simulink model "regler"  (Simulink 7.9)
settings: Solver=ode3  StartTime=0.0  StopTime=10  FixedStep=0.01  MaxStep=1e-3  RelTol=1e-3
PreLoadFcn:
  | l=0.23 %Achsenlänge in m
  | mc=0.5 %Masse Chassis in kg
  | mm=0.02 %Masse einzelner Motor in Kg
  | J=(l^2)*0.5*((1/12)*mc+mm)%Trägheitmoment rollen+nicken
  | Jg=(1/12)*mc*(l^2)+mm*4*(l/2)^2%trägheitsmoment gieren
  | tau=1/16.28; %zeitkonstante pt1-glied
  | k=2.064e+04; %proportionalitätsfaktor pt1glied
  | mi_wurz=-(sqrt(2)/2)*l/2; %initwerte
  | plu_wurz=(sqrt(2)/2)*l/2; %initwerte
  | mges=0.5 %Gesamtmasse in kg
  | %Drehmomentfunktion
  | %Funktion M(n) AUfstellen
  | kt=0.415*1e-2; %Nm/A
  | p1=[1.4 , 25000];
  | p2=[15.5 , 15000];
  | m=(p2(2)-p1(2))/(p2(1)-p1(1));
  | c=p1(2)-m*p1(1);
  | mm=kt/m;
  | cm=(-1)*c*mm;
  | %Propeller Funktion
  | faktor = 0.8895305;
  | exponent = 2.015137;
  | 
  | %regelparameter
  | kp_roll=0.75
  | tn_roll=1000
  | tv_roll=1.5
  | tp_roll=0.04
  | kp_v_roll=5.8571
  | kp_a_roll=0.0070
  | 
  | kp_nick=0.75
  | tn_nick=1000
  | tv_nick=1.5
  | tp_nick=0.04
  | kp_v_nick=5.8571
  | kp_a_nick=0.0070
  | 
  | kp_gier=0.75
  | tn_gier=1000
  | tv_gier=1.5
  | tp_gier=0.04
  | kp_v_gier=5.8571
  | kp_a_gier=0.0070
  | 
  | %Motor skalierungsfaktor
  | k_motor_out=1;
  | %maximaldrehzahl Motor
  | n_max=20000;
libraries: simulink x4, aerolibutil x4
settings Model: Creator=Flo  LastModifiedBy=Flo  TunableVars=exponent,faktor,k_motor_out,kp_a_gier,kp_a_nick,kp_a_roll,kp_gier,kp_nick,kp_roll,kp_v_gier,kp_v_nick,kp_v_roll,n_max,tn_gier,tn_nick,tn_roll,tp_gier,tp_nick,tp_roll,tv_gier,tv_nick,tv_roll  TunableVarsStorageClass=ExportedGlobal,ExportedGlobal,ExportedGlobal,ExportedGlobal,ExportedGlobal,ExportedGlobal,ExportedGlobal,ExportedGlobal,ExportedGlobal,ExportedGlobal,ExportedGlobal,ExportedGlobal,ExportedGlobal,ExportedGlobal,ExportedGlobal,ExportedGlobal,ExportedGlobal,ExportedGlobal,ExportedGlobal,ExportedGlobal,ExportedGlobal,ExportedGlobal  TunableVarsTypeQualifier=,,,,,,,,,,,,,,,,,,,,,
settings OptimizationCC: InlineParams=on  UseSpecifiedMinMax=on  EnableMemcpy=off  PassReuseOutputArgsAs=Individual arguments  OptimizeModelRefInitCode=on  LifeSpan=1
settings RTWCC: SystemTargetFile=ert.tlc  TemplateMakefile=ert_default_tmf  Description=Embedded Coder  ProcessScript=ert_make_rtw_hook  TargetLang=C++  RTWCompilerOptimization=On  CheckMdlBeforeBuild=Warning
settings CodeAppCC: IgnoreCustomStorageClasses=off
settings ERTTargetCC: CodeReplacementLibrary=C89/C90 (ANSI)  ERTMultiwordTypeDef=User defined  MultiwordLength=2048  GenerateSampleERTMain=on  SupportComplex=off  SupportContinuousTime=on  ERTCustomFileTemplate=example_file_process.tlc  GlobalDataDefinition=InSourceFile  DataDefinitionFile=.c  GlobalDataReference=InSourceFile  ConvertIfToSwitch=off  SuppressUnreachableDefaultCases=off  EnableUserReplacementTypes=on

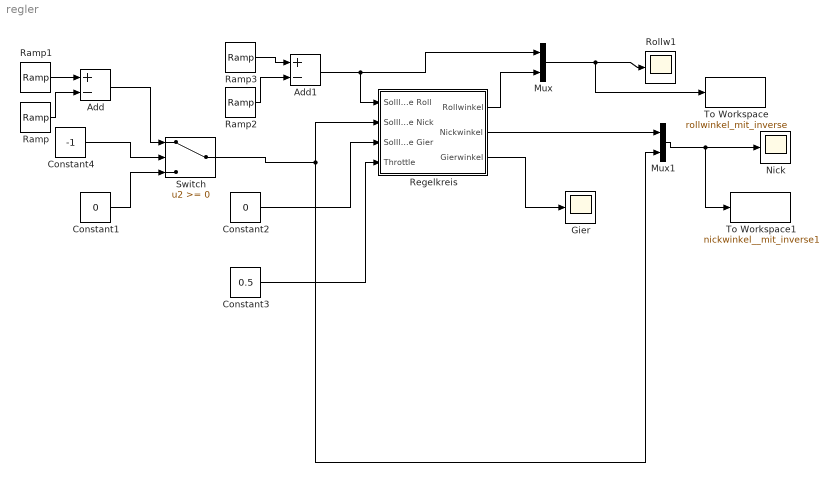
== system regler ==
  Add : Sum  Inputs=+-
  Add1 : Sum  Inputs=+-
  Constant1 : Constant  Value=0
  Constant2 : Constant  Value=0
  Constant3 : Constant  Value=0.5
  Constant4 : Constant  Value=-1
  Gier : Scope
      settings: YMin=0.05  YMax=0.275  SaveName=ScopeData25
  Mux : Mux  Inputs=2
  Mux1 : Mux  Inputs=2
  Nick : Scope
      settings: YMin=0.8  YMax=0.94  SaveName=ScopeData26
  Ramp : simulink/Sources/Ramp  slope=4  start=1.05  X0=0
  Ramp1 : simulink/Sources/Ramp  slope=4  start=1  X0=0
  Ramp2 : simulink/Sources/Ramp  slope=4  start=1.6  X0=0
  Ramp3 : simulink/Sources/Ramp  slope=4  start=1.5  X0=0
  Regelkreis : Subsystem
  Rollw1 : Scope
      settings: TimeRange=0.03425507699014805  YMin=0.5004659956947598  YMax=0.5014065398919517  SaveName=ScopeData2
  Switch : Switch
  To Workspace : ToWorkspace  VariableName=rollwinkel_mit_inverse  SampleTime=-1  SaveFormat=Timeseries
  To Workspace1 : ToWorkspace  VariableName=nickwinkel__mit_inverse1  SampleTime=-1  SaveFormat=Timeseries
  wires:
  Constant2/1 -> Regelkreis/3(Solllage Gier)
  Constant3/1 -> Regelkreis/4(Throttle)
  Regelkreis/1(Rollwinkel) -> Mux/2
  Regelkreis/3(Gierwinkel) -> Gier/1
  Ramp1/1 -> Add/1
  Ramp/1 -> Add/2
  Mux/1 -> Rollw1/1, To Workspace/1
  Add/1 -> Switch/1
  Constant4/1 -> Switch/2
  Ramp3/1 -> Add1/1
  Ramp2/1 -> Add1/2
  Switch/1 -> Regelkreis/2(Solllage Nick), Mux1/2
  Mux1/1 -> Nick/1, To Workspace1/1
  Regelkreis/2(Nickwinkel) -> Mux1/1
  Constant1/1 -> Switch/3
  Add1/1 -> Mux/1, Regelkreis/1(Solllage Roll)

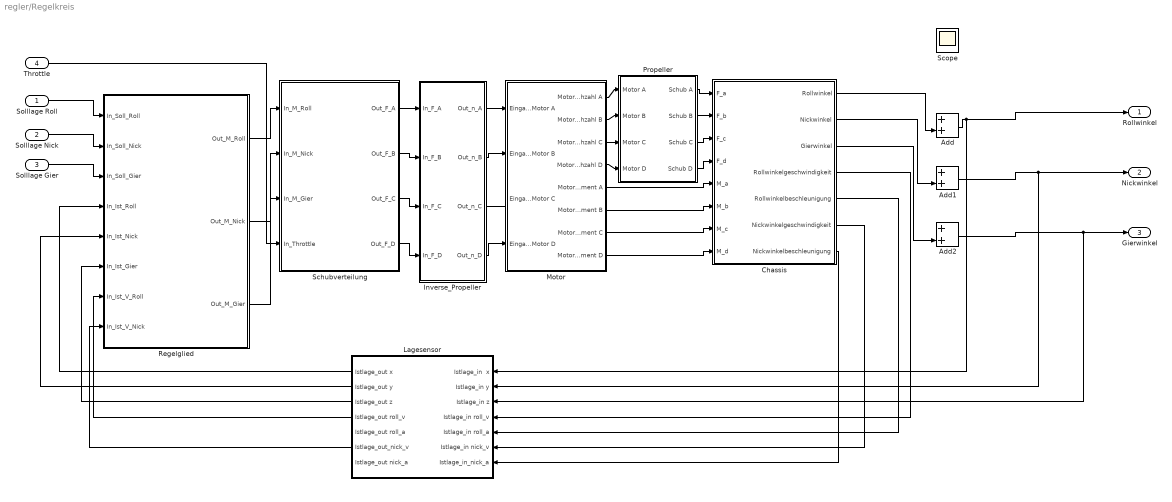
== system regler/Regelkreis ==
  Solllage Roll : Inport
  Solllage Nick : Inport  Port=2
  Solllage Gier : Inport  Port=3
  Throttle : Inport  Port=4
  Add : Sum
  Add1 : Sum
  Add2 : Sum
  Chassis : Subsystem
  Inverse_Propeller : Subsystem
  Lagesensor : Subsystem
  Motor : Subsystem
  Propeller : Subsystem
  Regelglied : Subsystem
  Schubverteilung : Subsystem
  Scope : Scope
      settings: SaveName=ScopeData5
  Rollwinkel : Outport
  Nickwinkel : Outport  Port=2
  Gierwinkel : Outport  Port=3
  wires:
  Motor/1(Motordrehzahl A) -> Propeller/1(Motor A)
  Motor/2(" Motordrehzahl B") -> Propeller/2(Motor B)
  Motor/3(Motordrehzahl C) -> Propeller/3(Motor C)
  Motor/4(Motordrehzahl D) -> Propeller/4(Motor D)
  Propeller/1(Schub A) -> Chassis/1(F_a)
  Propeller/2(Schub B) -> Chassis/2(F_b)
  Propeller/3(Schub C) -> Chassis/3(F_c)
  Propeller/4(Schub D) -> Chassis/4(F_d)
  Motor/5(Motormoment A) -> Chassis/5(M_a)
  Motor/6(" Motormoment B") -> Chassis/6(M_b)
  Motor/7(Motormoment C) -> Chassis/7(M_c)
  Motor/8(Motormoment D) -> Chassis/8(M_d)
  Solllage Roll/1 -> Regelglied/1(In_Soll_Roll)
  Solllage Nick/1 -> Regelglied/2(In_Soll_Nick)
  Solllage Gier/1 -> Regelglied/3(In_Soll_Gier)
  Lagesensor/1(Istlage_out x) -> Regelglied/4(In_Ist_Roll)
  Lagesensor/2(Istlage_out y) -> Regelglied/5(In_Ist_Nick)
  Lagesensor/3(Istlage_out z) -> Regelglied/6(In_Ist_Gier)
  Chassis/2(Nickwinkel) -> Add1/2
  Chassis/1(Rollwinkel) -> Add/2
  Chassis/3(Gierwinkel) -> Add2/2
  Add/1 -> Rollwinkel/1, Lagesensor/1(Istlage_in  x)
  Add1/1 -> Nickwinkel/1, Lagesensor/2(Istlage_in y)
  Add2/1 -> Gierwinkel/1, Lagesensor/3(Istlage_in z)
  ? -> Add1/1, Add2/1, Add/1, Scope/1
  Regelglied/1(Out_M_Roll) -> Schubverteilung/1(In_M_Roll)
  Regelglied/2(Out_M_Nick) -> Schubverteilung/2(In_M_Nick)
  Regelglied/3(Out_M_Gier) -> Schubverteilung/3(In_M_Gier)
  Chassis/4(Rollwinkelgeschwindigkeit) -> Lagesensor/4(Istlage_in roll_v)
  Lagesensor/4(Istlage_out roll_v) -> Regelglied/7(In_Ist_V_Roll)
  Chassis/5(Rollwinkelbeschleunigung) -> Lagesensor/5(Istlage_in roll_a)
  Chassis/6(Nickwinkelgeschwindigkeit) -> Lagesensor/6(Istlage_in nick_v)
  Chassis/7(Nickwinkelbeschleunigung) -> Lagesensor/7(Istlage_in_nick_a)
  Lagesensor/6(Istlage_out_nick_v) -> Regelglied/8(In_Ist_V_Nick)
  Schubverteilung/1(Out_F_A) -> Inverse_Propeller/1(In_F_A)
  Schubverteilung/2(Out_F_B) -> Inverse_Propeller/2(In_F_B)
  Schubverteilung/3(Out_F_C) -> Inverse_Propeller/3(In_F_C)
  Schubverteilung/4(Out_F_D) -> Inverse_Propeller/4(In_F_D)
  Inverse_Propeller/1(Out_n_A) -> Motor/1(Eingang Motor A)
  Inverse_Propeller/2(Out_n_B) -> Motor/2(Eingang Motor B)
  Inverse_Propeller/3(Out_n_C) -> Motor/3(Eingang Motor C)
  Inverse_Propeller/4(Out_n_D) -> Motor/4(Eingang Motor D)
  Throttle/1 -> Schubverteilung/4(In_Throttle)

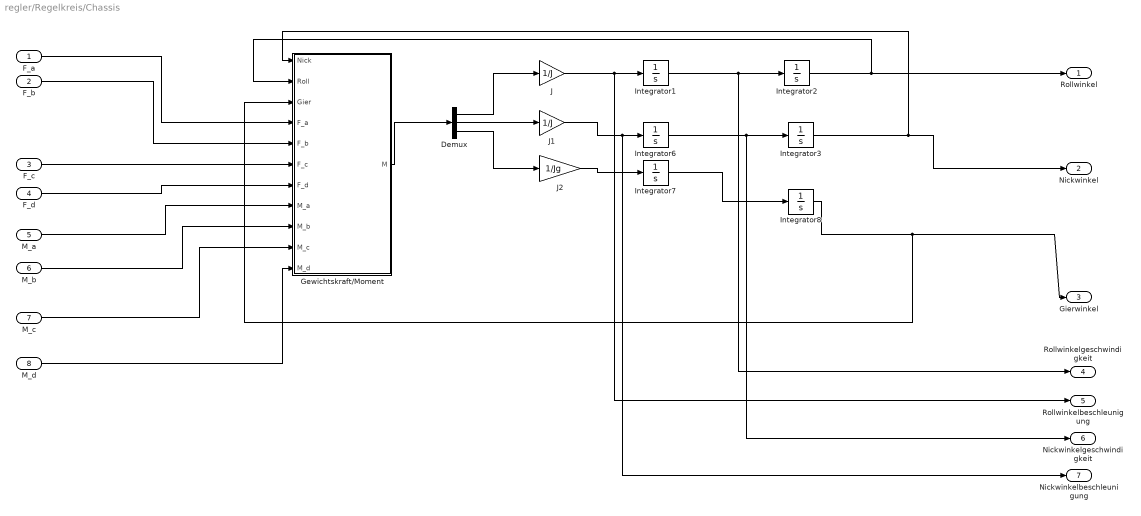
== system regler/Regelkreis/Chassis ==
  F_a : Inport
  F_b : Inport  Port=2
  F_c : Inport  Port=3
  F_d : Inport  Port=4
  M_a : Inport  Port=5
  M_b : Inport  Port=6
  M_c : Inport  Port=7
  M_d : Inport  Port=8
  Demux : Demux  Outputs=3
  Gewichtskraft/Moment : Subsystem
  Integrator{1..3,6..8} (6 alike) : Integrator
  J : Gain  Gain=1/J
  J1 : Gain  Gain=1/J
  J2 : Gain  Gain=1/Jg
  Rollwinkel : Outport
  Nickwinkel : Outport  Port=2
  Gierwinkel : Outport  Port=3
  Rollwinkelgeschwindigkeit : Outport  Port=4
  Rollwinkelbeschleunigung : Outport  Port=5
  Nickwinkelgeschwindigkeit : Outport  Port=6
  Nickwinkelbeschleunigung : Outport  Port=7
  wires:
  F_a/1 -> Gewichtskraft/Moment/4(F_a)
  F_b/1 -> Gewichtskraft/Moment/5(F_b)
  F_c/1 -> Gewichtskraft/Moment/6(F_c)
  F_d/1 -> Gewichtskraft/Moment/7(F_d)
  Gewichtskraft/Moment/1(M) -> Demux/1
  Demux/1 -> J/1
  Demux/2 -> J1/1
  Demux/3 -> J2/1
  J/1 -> Integrator1/1, Rollwinkelbeschleunigung/1
  Integrator1/1 -> Integrator2/1, Rollwinkelgeschwindigkeit/1
  Integrator2/1 -> Rollwinkel/1, Gewichtskraft/Moment/2(Roll)
  J1/1 -> Integrator6/1, Nickwinkelbeschleunigung/1
  Integrator6/1 -> Integrator3/1, Nickwinkelgeschwindigkeit/1
  Integrator3/1 -> Nickwinkel/1, Gewichtskraft/Moment/1(Nick)
  J2/1 -> Integrator7/1
  Integrator7/1 -> Integrator8/1
  Integrator8/1 -> Gierwinkel/1, Gewichtskraft/Moment/3(Gier)
  M_a/1 -> Gewichtskraft/Moment/8(M_a)
  M_b/1 -> Gewichtskraft/Moment/9(M_b)
  M_c/1 -> Gewichtskraft/Moment/10(M_c)
  M_d/1 -> Gewichtskraft/Moment/11(M_d)

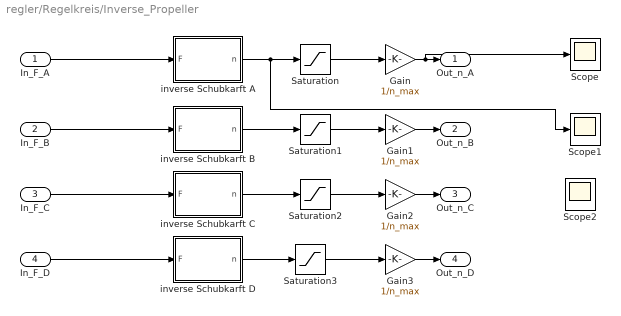
== system regler/Regelkreis/Inverse_Propeller ==
  In_F_A : Inport
  In_F_B : Inport  Port=2
  In_F_C : Inport  Port=3
  In_F_D : Inport  Port=4
  " inverse Schubkarft A" : Subsystem
  " inverse Schubkarft B" : Subsystem
  " inverse Schubkarft C" : Subsystem
  " inverse Schubkarft D" : Subsystem
  Gain{,1..3} (4 alike) : Gain  Gain=1/n_max
  Saturation{,1..3} (4 alike) : Saturate  UpperLimit=n_max  LowerLimit=0
  Scope : Scope
  Scope1 : Scope
      settings: SaveName=ScopeData4
  Scope2 : Scope
      settings: SaveName=ScopeData7
  Out_n_A : Outport
  Out_n_B : Outport  Port=2
  Out_n_C : Outport  Port=3
  Out_n_D : Outport  Port=4
  wires:
  " inverse Schubkarft A"/1(n) -> Saturation/1, Scope1/1
  " inverse Schubkarft B"/1(n) -> Saturation1/1
  " inverse Schubkarft C"/1(n) -> Saturation2/1
  " inverse Schubkarft D"/1(n) -> Saturation3/1
  In_F_A/1 -> " inverse Schubkarft A"/1(F)
  In_F_B/1 -> " inverse Schubkarft B"/1(F)
  In_F_C/1 -> " inverse Schubkarft C"/1(F)
  In_F_D/1 -> " inverse Schubkarft D"/1(F)
  Gain/1 -> Out_n_A/1, Scope/1
  Gain1/1 -> Out_n_B/1
  Gain2/1 -> Out_n_C/1
  Gain3/1 -> Out_n_D/1
  Saturation/1 -> Gain/1
  Saturation1/1 -> Gain1/1
  Saturation2/1 -> Gain2/1
  Saturation3/1 -> Gain3/1

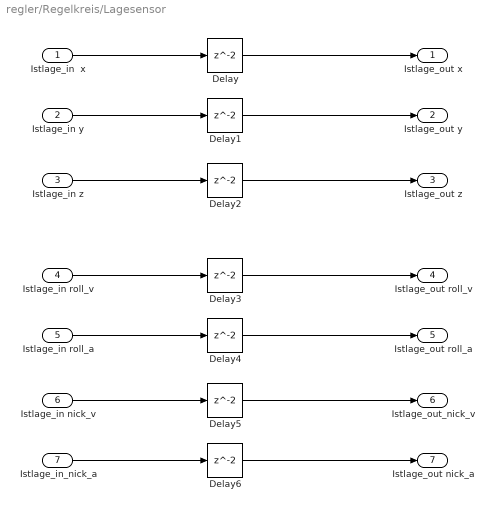
== system regler/Regelkreis/Lagesensor ==
  Istlage_in  x : Inport
  Istlage_in y : Inport  Port=2
  Istlage_in z : Inport  Port=3
  Istlage_in roll_v : Inport  Port=4
  Istlage_in roll_a : Inport  Port=5
  Istlage_in nick_v : Inport  Port=6
  Istlage_in_nick_a : Inport  Port=7
  Delay{,1..6} (7 alike) : Delay
  Istlage_out x : Outport
  Istlage_out y : Outport  Port=2
  Istlage_out z : Outport  Port=3
  Istlage_out roll_v : Outport  Port=4
  Istlage_out roll_a : Outport  Port=5
  Istlage_out_nick_v : Outport  Port=6
  Istlage_out nick_a : Outport  Port=7
  wires:
  Istlage_in  x/1 -> Delay/1
  Delay/1 -> Istlage_out x/1
  Istlage_in y/1 -> Delay1/1
  Delay2/1 -> Istlage_out z/1
  Istlage_in z/1 -> Delay2/1
  Delay1/1 -> Istlage_out y/1
  Istlage_in roll_v/1 -> Delay3/1
  Delay3/1 -> Istlage_out roll_v/1
  Istlage_in roll_a/1 -> Delay4/1
  Delay4/1 -> Istlage_out roll_a/1
  Istlage_in nick_v/1 -> Delay5/1
  Delay5/1 -> Istlage_out_nick_v/1
  Istlage_in_nick_a/1 -> Delay6/1
  Delay6/1 -> Istlage_out nick_a/1

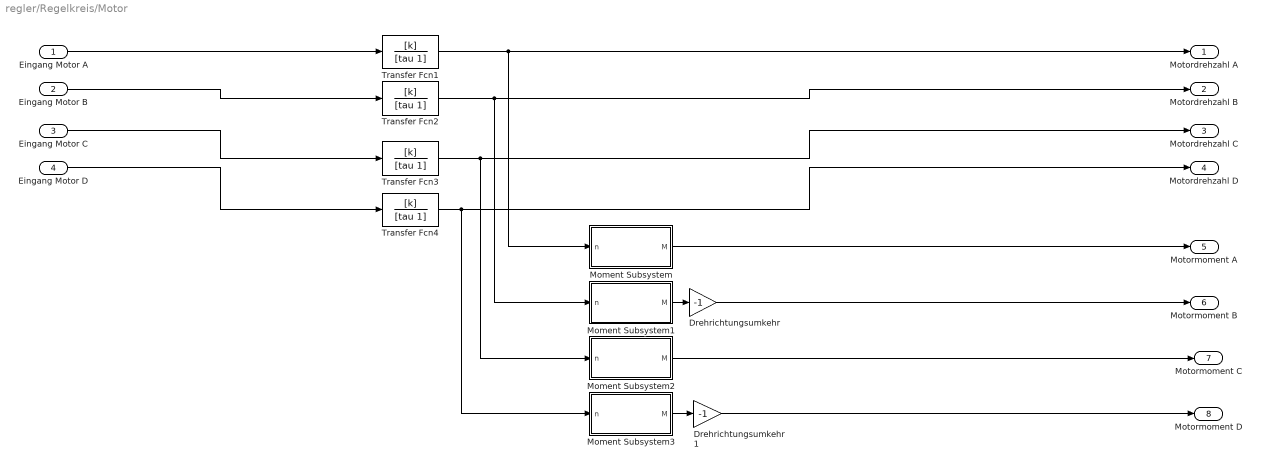
== system regler/Regelkreis/Motor ==
  Eingang Motor A : Inport
  Eingang Motor B : Inport  Port=2
  Eingang Motor C : Inport  Port=3
  Eingang Motor D : Inport  Port=4
  Drehrichtungsumkehr : Gain  Gain=-1
  Drehrichtungsumkehr1 : Gain  Gain=-1
  Moment Subsystem : Subsystem
  Moment Subsystem1 : Subsystem
  Moment Subsystem2 : Subsystem
  Moment Subsystem3 : Subsystem
  Transfer Fcn{1..4} (4 alike) : TransferFcn  Numerator=[k]  Denominator=[tau 1]
  Motordrehzahl A : Outport
  " Motordrehzahl B" : Outport  Port=2
  Motordrehzahl C : Outport  Port=3
  Motordrehzahl D : Outport  Port=4
  Motormoment A : Outport  Port=5
  " Motormoment B" : Outport  Port=6
  Motormoment C : Outport  Port=7
  Motormoment D : Outport  Port=8
  wires:
  Transfer Fcn1/1 -> Motordrehzahl A/1, Moment Subsystem/1(n)
  Transfer Fcn2/1 -> " Motordrehzahl B"/1, Moment Subsystem1/1(n)
  Transfer Fcn3/1 -> Motordrehzahl C/1, Moment Subsystem2/1(n)
  Transfer Fcn4/1 -> Motordrehzahl D/1, Moment Subsystem3/1(n)
  Moment Subsystem/1(M) -> Motormoment A/1
  Moment Subsystem1/1(M) -> Drehrichtungsumkehr/1
  Moment Subsystem3/1(M) -> Drehrichtungsumkehr1/1
  Moment Subsystem2/1(M) -> Motormoment C/1
  Drehrichtungsumkehr1/1 -> Motormoment D/1
  Drehrichtungsumkehr/1 -> " Motormoment B"/1
  Eingang Motor A/1 -> Transfer Fcn1/1
  Eingang Motor B/1 -> Transfer Fcn2/1
  Eingang Motor C/1 -> Transfer Fcn3/1
  Eingang Motor D/1 -> Transfer Fcn4/1

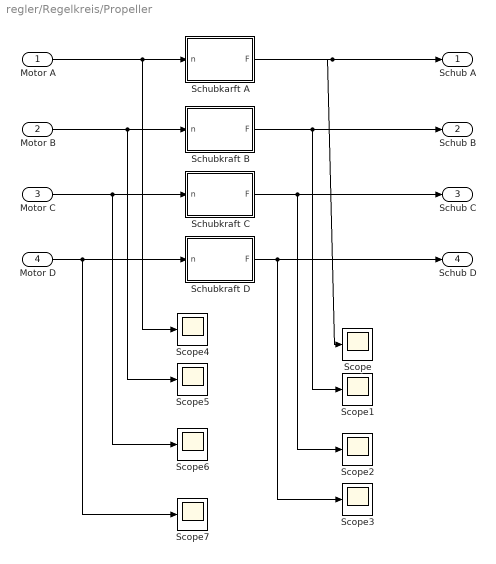
== system regler/Regelkreis/Propeller ==
  Motor A : Inport
  Motor B : Inport  Port=2
  Motor C : Inport  Port=3
  Motor D : Inport  Port=4
  Schubkarft A : Subsystem
  Schubkraft B : Subsystem
  Schubkraft C : Subsystem
  Schubkraft D : Subsystem
  Scope{,1..7} (8 alike) : Scope
      Scope settings: SaveName=ScopeData13
      Scope1 settings: SaveName=ScopeData14
      Scope2 settings: SaveName=ScopeData15
      Scope3 settings: SaveName=ScopeData16
      Scope4 settings: SaveName=ScopeData20
      Scope5 settings: SaveName=ScopeData21
      Scope6 settings: SaveName=ScopeData22
      Scope7 settings: SaveName=ScopeData23
  Schub A : Outport
  Schub B : Outport  Port=2
  Schub C : Outport  Port=3
  Schub D : Outport  Port=4
  wires:
  Motor A/1 -> Schubkarft A/1(n), Scope4/1
  Schubkarft A/1(F) -> Schub A/1, Scope/1
  Motor B/1 -> Schubkraft B/1(n), Scope5/1
  Schubkraft B/1(F) -> Schub B/1, Scope1/1
  Motor C/1 -> Schubkraft C/1(n), Scope6/1
  Schubkraft C/1(F) -> Schub C/1, Scope2/1
  Motor D/1 -> Schubkraft D/1(n), Scope7/1
  Schubkraft D/1(F) -> Schub D/1, Scope3/1

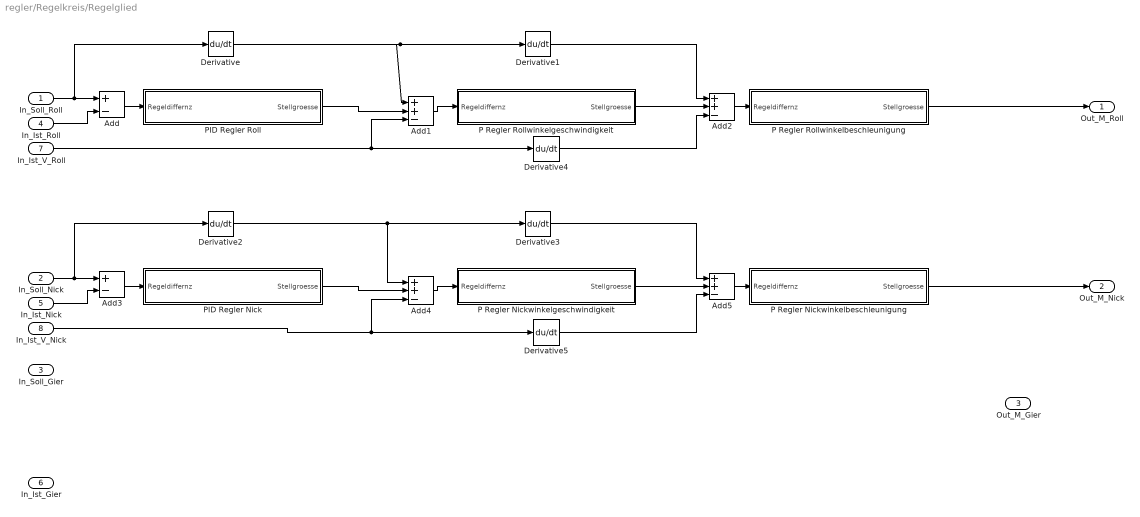
== system regler/Regelkreis/Regelglied ==
  In_Soll_Roll : Inport
  In_Soll_Nick : Inport  Port=2
  In_Soll_Gier : Inport  Port=3
  In_Ist_Roll : Inport  Port=4
  In_Ist_Nick : Inport  Port=5
  In_Ist_Gier : Inport  Port=6
  In_Ist_V_Roll : Inport  Port=7
  In_Ist_V_Nick : Inport  Port=8
  Add : Sum  Inputs=+-
  Add{1..2,4..5} (4 alike) : Sum  Inputs=++-
  Add3 : Sum  Inputs=+-
  Derivative{,1..5} (6 alike) : Derivative
  P Regler Nickwinkelbeschleunigung : Subsystem
  P Regler Nickwinkelgeschwindigkeit : Subsystem
  P Regler Rollwinkelbeschleunigung : Subsystem
  P Regler Rollwinkelgeschwindigkeit : Subsystem
  PID Regler Nick : Subsystem
  PID Regler Roll : Subsystem
  Out_M_Roll : Outport
  Out_M_Nick : Outport  Port=2
  Out_M_Gier : Outport  Port=3
  wires:
  In_Soll_Roll/1 -> Add/1, Derivative/1
  Add/1 -> PID Regler Roll/1(Regeldiffernz)
  In_Ist_Roll/1 -> Add/2
  Add1/1 -> P Regler Rollwinkelgeschwindigkeit/1(Regeldiffernz)
  Add2/1 -> P Regler Rollwinkelbeschleunigung/1(Regeldiffernz)
  P Regler Rollwinkelbeschleunigung/1(Stellgroesse) -> Out_M_Roll/1
  P Regler Rollwinkelgeschwindigkeit/1(Stellgroesse) -> Add2/2
  PID Regler Roll/1(Stellgroesse) -> Add1/2
  Derivative/1 -> Derivative1/1, Add1/1
  In_Soll_Nick/1 -> Derivative2/1, Add3/1
  Add3/1 -> PID Regler Nick/1(Regeldiffernz)
  In_Ist_Nick/1 -> Add3/2
  Add4/1 -> P Regler Nickwinkelgeschwindigkeit/1(Regeldiffernz)
  Add5/1 -> P Regler Nickwinkelbeschleunigung/1(Regeldiffernz)
  P Regler Nickwinkelbeschleunigung/1(Stellgroesse) -> Out_M_Nick/1
  P Regler Nickwinkelgeschwindigkeit/1(Stellgroesse) -> Add5/2
  PID Regler Nick/1(Stellgroesse) -> Add4/2
  Derivative2/1 -> Derivative3/1, Add4/1
  Derivative1/1 -> Add2/1
  Derivative4/1 -> Add2/3
  In_Ist_V_Roll/1 -> Derivative4/1, Add1/3
  Derivative3/1 -> Add5/1
  Derivative5/1 -> Add5/3
  In_Ist_V_Nick/1 -> Derivative5/1, Add4/3

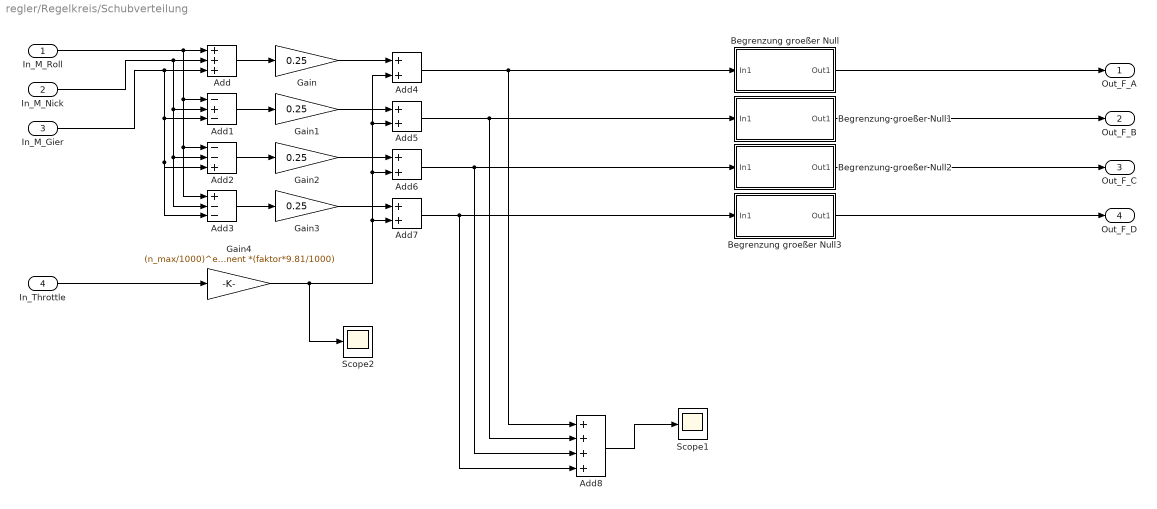
== system regler/Regelkreis/Schubverteilung ==
  In_M_Roll : Inport  OutDataTypeStr=double  LockScale=on
  In_M_Nick : Inport  Port=2  OutDataTypeStr=double
  In_M_Gier : Inport  Port=3  OutDataTypeStr=double
  In_Throttle : Inport  Port=4  OutDataTypeStr=double
  Add : Sum  Inputs=+++  OutDataTypeStr=double
  Add1 : Sum  Inputs=-+-  OutDataTypeStr=double
  Add2 : Sum  Inputs=--+  OutDataTypeStr=double
  Add3 : Sum  Inputs=+--  OutDataTypeStr=double
  Add{4..7} (4 alike) : Sum
  Add8 : Sum  Inputs=++++  AccumDataTypeStr=double  OutDataTypeStr=double
  Begrenzung groeßer Null : Subsystem
  Begrenzung groeßer Null1 : Subsystem
  Begrenzung groeßer Null2 : Subsystem
  Begrenzung groeßer Null3 : Subsystem
  Gain{,1..3} (4 alike) : Gain  Gain=0.25  OutDataTypeStr=double
  Gain4 : Gain  Gain=(n_max/1000)^exponent *(faktor*9.81/1000)  OutDataTypeStr=double
  Scope1 : Scope
      settings: YMin=1.9  YMax=2.1  SaveName=ScopeData3
  Scope2 : Scope
      settings: YMin=1.9  YMax=2.1  SaveName=ScopeData6
  Out_F_A : Outport  OutDataTypeStr=double
  Out_F_B : Outport  Port=2  OutDataTypeStr=double
  Out_F_C : Outport  Port=3  OutDataTypeStr=double
  Out_F_D : Outport  Port=4  OutDataTypeStr=double
  wires:
  In_M_Roll/1 -> Add/1, Add1/1, Add2/1, Add3/1
  In_M_Nick/1 -> Add/2, Add1/2, Add2/2, Add3/2
  In_M_Gier/1 -> Add/3, Add1/3, Add2/3, Add3/3
  Add/1 -> Gain/1
  Add1/1 -> Gain1/1
  Add2/1 -> Gain2/1
  Add3/1 -> Gain3/1
  Add8/1 -> Scope1/1
  Begrenzung groeßer Null/1(Out1) -> Out_F_A/1
  Begrenzung groeßer Null1/1(Out1) -> Out_F_B/1
  Begrenzung groeßer Null2/1(Out1) -> Out_F_C/1
  Begrenzung groeßer Null3/1(Out1) -> Out_F_D/1
  Gain/1 -> Add4/1
  Gain1/1 -> Add5/1
  Gain2/1 -> Add6/1
  Gain3/1 -> Add7/1
  In_Throttle/1 -> Gain4/1
  Add4/1 -> Begrenzung groeßer Null/1(In1), Add8/1
  Add5/1 -> Begrenzung groeßer Null1/1(In1), Add8/2
  Add6/1 -> Begrenzung groeßer Null2/1(In1), Add8/3
  Add7/1 -> Begrenzung groeßer Null3/1(In1), Add8/4
  Gain4/1 -> Add4/2, Add5/2, Add6/2, Add7/2, Scope2/1

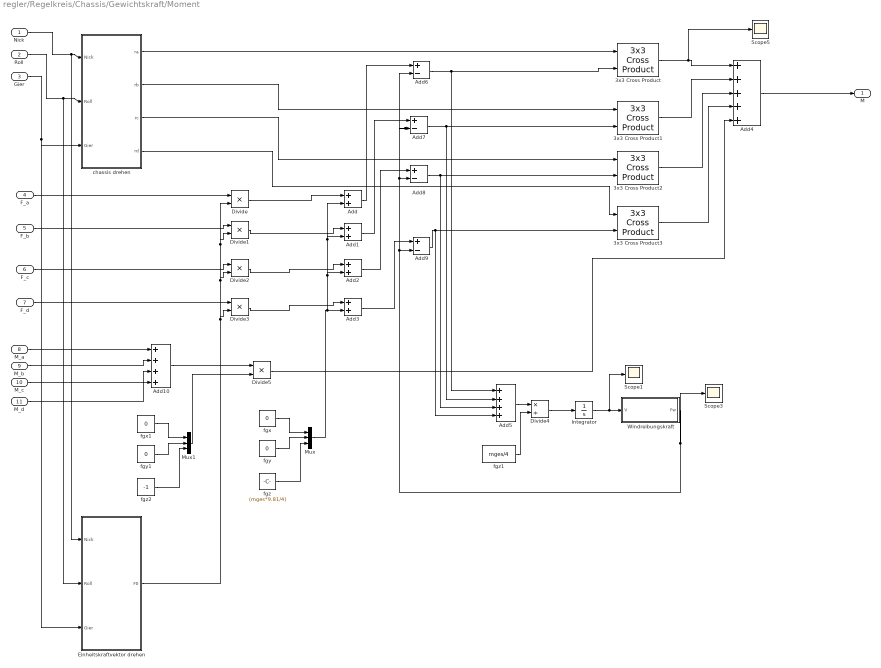
== system regler/Regelkreis/Chassis/Gewichtskraft/Moment ==
  Nick : Inport
  Roll : Inport  Port=2
  Gier : Inport  Port=3
  F_a : Inport  Port=4
  F_b : Inport  Port=5
  F_c : Inport  Port=6
  F_d : Inport  Port=7
  M_a : Inport  Port=8
  M_b : Inport  Port=9
  M_c : Inport  Port=10
  M_d : Inport  Port=11
  3x3 Cross Product{,1..3} (4 alike) : aerolibutil/3x3 Cross Product
  Add{,1..3} (4 alike) : Sum
  Add10 : Sum  Inputs=++++
  Add4 : Sum  Inputs=+++++
  Add5 : Sum  Inputs=++++
  Add{6..9} (4 alike) : Sum  Inputs=+-
  Divide{,1..3,5} (5 alike) : Product  Inputs=**
  Divide4 : Product  Inputs=*/
  Einheitskraftvektor drehen : Subsystem
  Integrator : Integrator
  Mux : Mux  Inputs=3
  Mux1 : Mux  Inputs=3
  Scope1 : Scope
      settings: TimeRange=2.186311787072243  YMin=-3.46945e-18  YMax=0.13  SaveName=ScopeData9
  Scope3 : Scope
      settings: TimeRange=2.186311787072243  YMin=-3.46945e-18  YMax=0.13
  Scope5 : Scope
      settings: SaveName=ScopeData17
  Windreibungskraft : Subsystem
  chassis drehen : Subsystem
  fgx : Constant  Value=0
  fgx1 : Constant  Value=0
  fgy : Constant  Value=0
  fgy1 : Constant  Value=0
  fgz : Constant  Value=(mges*9.81/4)
  fgz1 : Constant  Value=mges/4
  fgz2 : Constant  Value=-1
  M : Outport
  wires:
  F_a/1 -> Divide/1
  F_b/1 -> Divide1/1
  F_c/1 -> Divide2/1
  F_d/1 -> Divide3/1
  Nick/1 -> chassis drehen/1(Nick), Einheitskraftvektor drehen/1(Nick)
  Roll/1 -> chassis drehen/2(Roll), Einheitskraftvektor drehen/2(Roll)
  Gier/1 -> chassis drehen/3(Gier), Einheitskraftvektor drehen/3(Gier)
  Einheitskraftvektor drehen/1(F0) -> Divide/2, Divide1/2, Divide2/2, Divide3/2
  chassis drehen/1(ra) -> 3x3 Cross Product/1
  chassis drehen/2(rb) -> 3x3 Cross Product1/1
  chassis drehen/3(rc) -> 3x3 Cross Product2/1
  chassis drehen/4(rd) -> 3x3 Cross Product3/1
  fgx/1 -> Mux/1
  fgy/1 -> Mux/2
  fgz/1 -> Mux/3
  Mux/1 -> Add3/2, Add/2, Add1/2, Add2/2
  Divide/1 -> Add/1
  Divide2/1 -> Add2/1
  Divide1/1 -> Add1/1
  Divide3/1 -> Add3/1
  Add/1 -> Add6/1
  Add1/1 -> Add7/1
  Add2/1 -> Add8/1
  Add3/1 -> Add9/1
  3x3 Cross Product/1 -> Add4/1, Scope5/1
  3x3 Cross Product1/1 -> Add4/2
  3x3 Cross Product2/1 -> Add4/3
  3x3 Cross Product3/1 -> Add4/4
  Add4/1 -> M/1
  Add5/1 -> Divide4/1
  fgz1/1 -> Divide4/2
  Divide4/1 -> Integrator/1
  Integrator/1 -> Windreibungskraft/1(V), Scope1/1
  Add6/1 -> 3x3 Cross Product/2, Add5/1
  Add7/1 -> 3x3 Cross Product1/2, Add5/2
  Add8/1 -> 3x3 Cross Product2/2, Add5/3
  Add9/1 -> Add5/4, 3x3 Cross Product3/2
  Windreibungskraft/1(Fw) -> Add6/2, Add7/2, Add8/2, Add9/2, Scope3/1
  M_a/1 -> Add10/1
  M_b/1 -> Add10/2
  M_c/1 -> Add10/3
  M_d/1 -> Add10/4
  fgx1/1 -> Mux1/1
  fgy1/1 -> Mux1/2
  fgz2/1 -> Mux1/3
  Mux1/1 -> Divide5/2
  Add10/1 -> Divide5/1
  Divide5/1 -> Add4/5

== system regler/Regelkreis/Inverse_Propeller/ inverse Schubkarft A ==
  F : Inport
  Constant2 : Constant  Value=faktor*9.81/1000
  Constant3 : Constant  Value=1/exponent
  Divide1 : Product  Inputs=*/
  Gain : Gain  Gain=1000
  Math Function1 : Math  Operator=pow  SaturateOnIntegerOverflow=on
  n : Outport
  wires:
  F/1 -> Divide1/1
  Constant2/1 -> Divide1/2
  Divide1/1 -> Math Function1/1
  Constant3/1 -> Math Function1/2
  Math Function1/1 -> Gain/1
  Gain/1 -> n/1

== system regler/Regelkreis/Inverse_Propeller/ inverse Schubkarft B ==
  F : Inport
  Constant2 : Constant  Value=faktor*9.81/1000
  Constant3 : Constant  Value=1/exponent
  Divide1 : Product  Inputs=*/
  Gain : Gain  Gain=1000
  Math Function1 : Math  Operator=pow  SaturateOnIntegerOverflow=on
  n : Outport
  wires:
  Gain/1 -> n/1
  Math Function1/1 -> Gain/1
  Constant3/1 -> Math Function1/2
  Divide1/1 -> Math Function1/1
  Constant2/1 -> Divide1/2
  F/1 -> Divide1/1

== system regler/Regelkreis/Inverse_Propeller/ inverse Schubkarft C ==
  F : Inport
  Constant2 : Constant  Value=faktor*9.81/1000
  Constant3 : Constant  Value=1/exponent
  Divide1 : Product  Inputs=*/
  Gain : Gain  Gain=1000
  Math Function1 : Math  Operator=pow  SaturateOnIntegerOverflow=on
  n : Outport
  wires:
  F/1 -> Divide1/1
  Constant2/1 -> Divide1/2
  Divide1/1 -> Math Function1/1
  Constant3/1 -> Math Function1/2
  Math Function1/1 -> Gain/1
  Gain/1 -> n/1

== system regler/Regelkreis/Inverse_Propeller/ inverse Schubkarft D ==
  F : Inport
  Constant2 : Constant  Value=faktor*9.81/1000
  Constant3 : Constant  Value=1/exponent
  Divide1 : Product  Inputs=*/
  Gain : Gain  Gain=1000
  Math Function1 : Math  Operator=pow  SaturateOnIntegerOverflow=on
  n : Outport
  wires:
  Gain/1 -> n/1
  Math Function1/1 -> Gain/1
  Constant3/1 -> Math Function1/2
  Divide1/1 -> Math Function1/1
  Constant2/1 -> Divide1/2
  F/1 -> Divide1/1

== system regler/Regelkreis/Motor/Moment Subsystem ==
  n : Inport
  If : If
  Merge : Merge  InitialOutput=0
  n<1 : Subsystem  TreatAsAtomicUnit=on
  n>0 : Subsystem  TreatAsAtomicUnit=on
  M : Outport
  wires:
  n/1 -> If/1, n>0/1(n)
  If/1 -> n>0/Action
  If/2 -> n<1/Action
  n>0/1(M) -> Merge/1
  n<1/1(M) -> Merge/2
  Merge/1 -> M/1

== system regler/Regelkreis/Motor/Moment Subsystem1 ==
  n : Inport
  If : If
  Merge : Merge  InitialOutput=0
  n<1 : Subsystem  TreatAsAtomicUnit=on
  n>0 : Subsystem  TreatAsAtomicUnit=on
  M : Outport
  wires:
  Merge/1 -> M/1
  n<1/1(M) -> Merge/2
  n>0/1(M) -> Merge/1
  If/2 -> n<1/Action
  If/1 -> n>0/Action
  n/1 -> n>0/1(n), If/1

== system regler/Regelkreis/Motor/Moment Subsystem2 ==
  n : Inport
  If : If
  Merge : Merge  InitialOutput=0
  n<1 : Subsystem  TreatAsAtomicUnit=on
  n>0 : Subsystem  TreatAsAtomicUnit=on
  M : Outport
  wires:
  n/1 -> If/1, n>0/1(n)
  If/1 -> n>0/Action
  If/2 -> n<1/Action
  n>0/1(M) -> Merge/1
  n<1/1(M) -> Merge/2
  Merge/1 -> M/1

== system regler/Regelkreis/Motor/Moment Subsystem3 ==
  n : Inport
  If : If
  Merge : Merge  InitialOutput=0
  n<1 : Subsystem  TreatAsAtomicUnit=on
  n>0 : Subsystem  TreatAsAtomicUnit=on
  M : Outport
  wires:
  Merge/1 -> M/1
  n<1/1(M) -> Merge/2
  n>0/1(M) -> Merge/1
  If/2 -> n<1/Action
  If/1 -> n>0/Action
  n/1 -> n>0/1(n), If/1

== system regler/Regelkreis/Propeller/Schubkarft A ==
  n : Inport
  Constant : Constant  Value=1000
  Constant1 : Constant  Value=exponent
  Divide : Product  Inputs=*/
  Gain : Gain  Gain=faktor*9.81/1000
  Math Function : Math  Operator=pow  SaturateOnIntegerOverflow=on
  F : Outport
  wires:
  n/1 -> Divide/1
  Constant/1 -> Divide/2
  Divide/1 -> Math Function/1
  Constant1/1 -> Math Function/2
  Math Function/1 -> Gain/1
  Gain/1 -> F/1

== system regler/Regelkreis/Propeller/Schubkraft B ==
  n : Inport
  Constant : Constant  Value=1000
  Constant1 : Constant  Value=exponent
  Divide : Product  Inputs=*/
  Gain : Gain  Gain=faktor*9.81/1000
  Math Function : Math  Operator=pow  SaturateOnIntegerOverflow=on
  F : Outport
  wires:
  Gain/1 -> F/1
  Math Function/1 -> Gain/1
  Constant1/1 -> Math Function/2
  Divide/1 -> Math Function/1
  Constant/1 -> Divide/2
  n/1 -> Divide/1

== system regler/Regelkreis/Propeller/Schubkraft C ==
  n : Inport
  Constant : Constant  Value=1000
  Constant1 : Constant  Value=exponent
  Divide : Product  Inputs=*/
  Gain : Gain  Gain=faktor*9.81/1000
  Math Function : Math  Operator=pow  SaturateOnIntegerOverflow=on
  F : Outport
  wires:
  n/1 -> Divide/1
  Constant/1 -> Divide/2
  Divide/1 -> Math Function/1
  Constant1/1 -> Math Function/2
  Math Function/1 -> Gain/1
  Gain/1 -> F/1

== system regler/Regelkreis/Propeller/Schubkraft D ==
  n : Inport
  Constant : Constant  Value=1000
  Constant1 : Constant  Value=exponent
  Divide : Product  Inputs=*/
  Gain : Gain  Gain=faktor*9.81/1000
  Math Function : Math  Operator=pow  SaturateOnIntegerOverflow=on
  F : Outport
  wires:
  Gain/1 -> F/1
  Math Function/1 -> Gain/1
  Constant1/1 -> Math Function/2
  Divide/1 -> Math Function/1
  Constant/1 -> Divide/2
  n/1 -> Divide/1

== system regler/Regelkreis/Regelglied/P Regler Nickwinkelbeschleunigung ==
  Regeldiffernz : Inport
  Gain : Gain  Gain=kp_a_nick
  Stellgroesse : Outport
  wires:
  Gain/1 -> Stellgroesse/1
  Regeldiffernz/1 -> Gain/1

== system regler/Regelkreis/Regelglied/P Regler Nickwinkelgeschwindigkeit ==
  Regeldiffernz : Inport
  Gain : Gain  Gain=kp_v_nick
  Stellgroesse : Outport
  wires:
  Gain/1 -> Stellgroesse/1
  Regeldiffernz/1 -> Gain/1

== system regler/Regelkreis/Regelglied/P Regler Rollwinkelbeschleunigung ==
  Regeldiffernz : Inport
  Gain : Gain  Gain=kp_a_roll
  Stellgroesse : Outport
  wires:
  Regeldiffernz/1 -> Gain/1
  Gain/1 -> Stellgroesse/1

== system regler/Regelkreis/Regelglied/P Regler Rollwinkelgeschwindigkeit ==
  Regeldiffernz : Inport
  Gain : Gain  Gain=kp_v_roll
  Stellgroesse : Outport
  wires:
  Regeldiffernz/1 -> Gain/1
  Gain/1 -> Stellgroesse/1

== system regler/Regelkreis/Regelglied/PID Regler Nick ==
  Regeldiffernz : Inport
  Add : Sum  Inputs=+++
  D-Anteil : TransferFcn  Numerator=[tv_nick 0]  Denominator=[tp_nick 1]
  Gain : Gain  Gain=kp_nick
  I-Anteil : TransferFcn  Denominator=[tn_nick 0]
  Stellgroesse : Outport
  wires:
  Gain/1 -> Add/1
  D-Anteil/1 -> Add/3
  I-Anteil/1 -> Add/2
  Regeldiffernz/1 -> D-Anteil/1, I-Anteil/1, Gain/1
  Add/1 -> Stellgroesse/1

== system regler/Regelkreis/Regelglied/PID Regler Roll ==
  Regeldiffernz : Inport
  Add : Sum  Inputs=+++
  D-Anteil : TransferFcn  Numerator=[tv_roll 0]  Denominator=[tp_roll 1]
  Gain : Gain  Gain=kp_roll
  I-Anteil : TransferFcn  Denominator=[tn_roll 0]
  Stellgroesse : Outport
  wires:
  Add/1 -> Stellgroesse/1
  Regeldiffernz/1 -> Gain/1, I-Anteil/1, D-Anteil/1
  I-Anteil/1 -> Add/2
  D-Anteil/1 -> Add/3
  Gain/1 -> Add/1

== system regler/Regelkreis/Schubverteilung/Begrenzung groeßer Null ==
  In1 : Inport
  If : If  IfExpression=u1 >= 0
  If Action Subsystem : Subsystem  TreatAsAtomicUnit=on
  If Action Subsystem1 : Subsystem  TreatAsAtomicUnit=on
  Merge : Merge  InitialOutput=0
  Out1 : Outport
  wires:
  In1/1 -> If/1, If Action Subsystem/1(In1)
  If/1 -> If Action Subsystem/Action
  If/2 -> If Action Subsystem1/Action
  Merge/1 -> Out1/1
  If Action Subsystem/1(Out1) -> Merge/1
  If Action Subsystem1/1(Out1) -> Merge/2

== system regler/Regelkreis/Schubverteilung/Begrenzung groeßer Null1 ==
  In1 : Inport
  If : If  IfExpression=u1 >= 0
  If Action Subsystem : Subsystem  TreatAsAtomicUnit=on
  If Action Subsystem1 : Subsystem  TreatAsAtomicUnit=on
  Merge : Merge  InitialOutput=0
  Out1 : Outport
  wires:
  If Action Subsystem1/1(Out1) -> Merge/2
  If Action Subsystem/1(Out1) -> Merge/1
  Merge/1 -> Out1/1
  If/2 -> If Action Subsystem1/Action
  If/1 -> If Action Subsystem/Action
  In1/1 -> If Action Subsystem/1(In1), If/1

== system regler/Regelkreis/Schubverteilung/Begrenzung groeßer Null2 ==
  In1 : Inport
  If : If  IfExpression=u1 >= 0
  If Action Subsystem : Subsystem  TreatAsAtomicUnit=on
  If Action Subsystem1 : Subsystem  TreatAsAtomicUnit=on
  Merge : Merge  InitialOutput=0
  Out1 : Outport
  wires:
  In1/1 -> If/1, If Action Subsystem/1(In1)
  If/1 -> If Action Subsystem/Action
  If/2 -> If Action Subsystem1/Action
  Merge/1 -> Out1/1
  If Action Subsystem/1(Out1) -> Merge/1
  If Action Subsystem1/1(Out1) -> Merge/2

== system regler/Regelkreis/Schubverteilung/Begrenzung groeßer Null3 ==
  In1 : Inport
  If : If  IfExpression=u1 >= 0
  If Action Subsystem : Subsystem  TreatAsAtomicUnit=on
  If Action Subsystem1 : Subsystem  TreatAsAtomicUnit=on
  Merge : Merge  InitialOutput=0
  Out1 : Outport
  wires:
  If Action Subsystem1/1(Out1) -> Merge/2
  If Action Subsystem/1(Out1) -> Merge/1
  Merge/1 -> Out1/1
  If/2 -> If Action Subsystem1/Action
  If/1 -> If Action Subsystem/Action
  In1/1 -> If Action Subsystem/1(In1), If/1

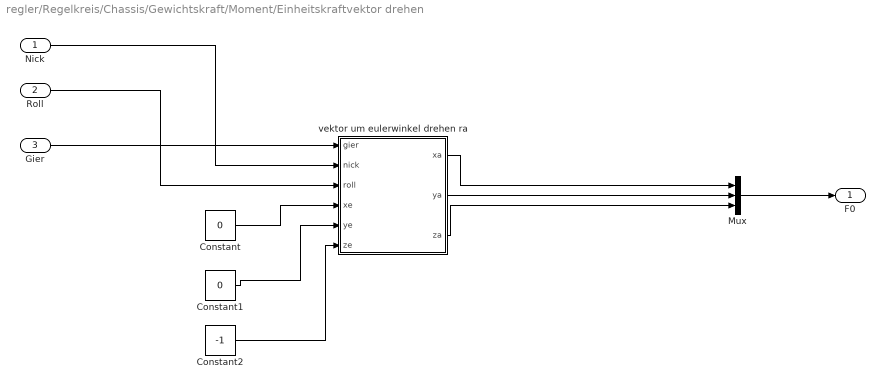
== system regler/Regelkreis/Chassis/Gewichtskraft/Moment/Einheitskraftvektor drehen ==
  Nick : Inport
  Roll : Inport  Port=2
  Gier : Inport  Port=3
  Constant : Constant  Value=0
  Constant1 : Constant  Value=0
  Constant2 : Constant  Value=-1
  Mux : Mux  Inputs=3
  vektor um eulerwinkel drehen ra : MATLAB Function  TreatAsAtomicUnit=on
  F0 : Outport
  wires:
  Gier/1 -> vektor um eulerwinkel drehen ra/1(gier)
  Roll/1 -> vektor um eulerwinkel drehen ra/3(roll)
  Nick/1 -> vektor um eulerwinkel drehen ra/2(nick)
  vektor um eulerwinkel drehen ra/3(za) -> Mux/3
  vektor um eulerwinkel drehen ra/2(ya) -> Mux/2
  vektor um eulerwinkel drehen ra/1(xa) -> Mux/1
  Mux/1 -> F0/1
  Constant/1 -> vektor um eulerwinkel drehen ra/4(xe)
  Constant1/1 -> vektor um eulerwinkel drehen ra/5(ye)
  Constant2/1 -> vektor um eulerwinkel drehen ra/6(ze)

== system regler/Regelkreis/Chassis/Gewichtskraft/Moment/Windreibungskraft ==
  V : Inport
  Constant : Constant  Value=0.5
  Cw-Wert : Constant  Value=2*0.01*l
  Divide : Product  Inputs=**
  Divide1 : Product  Inputs=*****
  Fläche : Constant  Value=2*0.01*l
  Luftdichte : Constant  Value=1.2041
  Fw : Outport
  wires:
  V/1 -> Divide/1, Divide/2
  Divide/1 -> Divide1/1
  Constant/1 -> Divide1/2
  Luftdichte/1 -> Divide1/3
  Fläche/1 -> Divide1/4
  Cw-Wert/1 -> Divide1/5
  Divide1/1 -> Fw/1

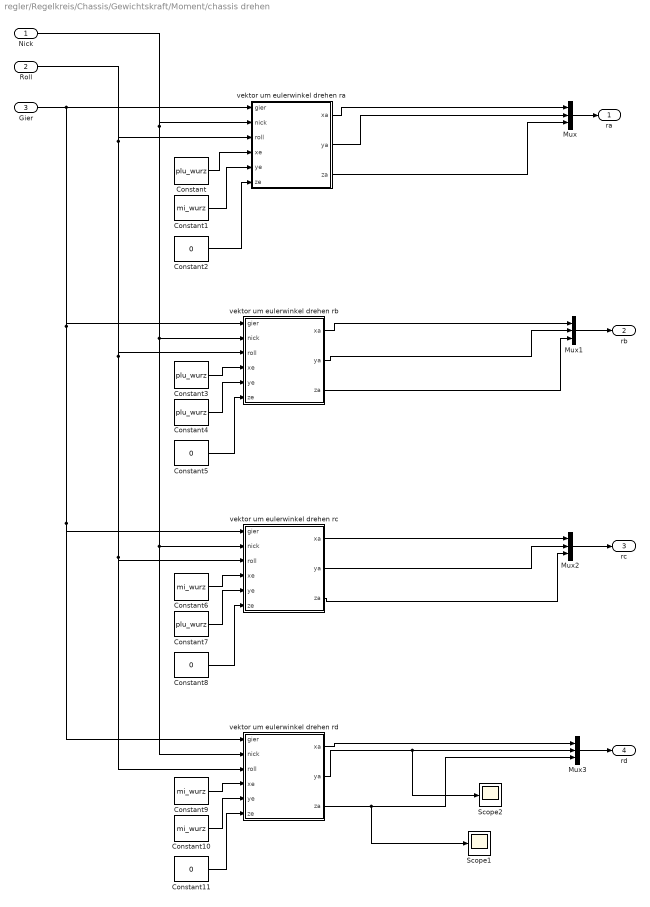
== system regler/Regelkreis/Chassis/Gewichtskraft/Moment/chassis drehen ==
  Nick : Inport
  Roll : Inport  Port=2
  Gier : Inport  Port=3
  Constant{,3..4,7} (4 alike) : Constant  Value=plu_wurz
  Constant{1,6,9..10} (4 alike) : Constant  Value=mi_wurz
  Constant{2,5,8,11} (4 alike) : Constant  Value=0
  Mux{,1..3} (4 alike) : Mux  Inputs=3
  Scope1 : Scope
      settings: SaveName=ScopeData18
  Scope2 : Scope
      settings: SaveName=ScopeData19
  vektor um eulerwinkel drehen ra : MATLAB Function  TreatAsAtomicUnit=on
  vektor um eulerwinkel drehen rb : MATLAB Function  TreatAsAtomicUnit=on
  vektor um eulerwinkel drehen rc : MATLAB Function  TreatAsAtomicUnit=on
  vektor um eulerwinkel drehen rd : MATLAB Function  TreatAsAtomicUnit=on
  ra : Outport
  rb : Outport  Port=2
  rc : Outport  Port=3
  rd : Outport  Port=4
  wires:
  vektor um eulerwinkel drehen rd/1(xa) -> Mux3/1
  vektor um eulerwinkel drehen rd/2(ya) -> Mux3/2, Scope2/1
  vektor um eulerwinkel drehen rc/1(xa) -> Mux2/1
  vektor um eulerwinkel drehen rc/2(ya) -> Mux2/2
  vektor um eulerwinkel drehen rc/3(za) -> Mux2/3
  vektor um eulerwinkel drehen rb/1(xa) -> Mux1/1
  vektor um eulerwinkel drehen rb/2(ya) -> Mux1/2
  vektor um eulerwinkel drehen rb/3(za) -> Mux1/3
  vektor um eulerwinkel drehen ra/1(xa) -> Mux/1
  vektor um eulerwinkel drehen ra/2(ya) -> Mux/2
  vektor um eulerwinkel drehen ra/3(za) -> Mux/3
  Nick/1 -> vektor um eulerwinkel drehen rd/2(nick), vektor um eulerwinkel drehen rc/2(nick), vektor um eulerwinkel drehen rb/2(nick), vektor um eulerwinkel drehen ra/2(nick)
  Roll/1 -> vektor um eulerwinkel drehen rd/3(roll), vektor um eulerwinkel drehen rc/3(roll), vektor um eulerwinkel drehen rb/3(roll), vektor um eulerwinkel drehen ra/3(roll)
  Gier/1 -> vektor um eulerwinkel drehen rd/1(gier), vektor um eulerwinkel drehen rc/1(gier), vektor um eulerwinkel drehen rb/1(gier), vektor um eulerwinkel drehen ra/1(gier)
  Mux1/1 -> rb/1
  Mux2/1 -> rc/1
  Mux3/1 -> rd/1
  Mux/1 -> ra/1
  vektor um eulerwinkel drehen rd/3(za) -> Mux3/3, Scope1/1
  Constant/1 -> vektor um eulerwinkel drehen ra/4(xe)
  Constant1/1 -> vektor um eulerwinkel drehen ra/5(ye)
  Constant2/1 -> vektor um eulerwinkel drehen ra/6(ze)
  Constant3/1 -> vektor um eulerwinkel drehen rb/4(xe)
  Constant4/1 -> vektor um eulerwinkel drehen rb/5(ye)
  Constant5/1 -> vektor um eulerwinkel drehen rb/6(ze)
  Constant6/1 -> vektor um eulerwinkel drehen rc/4(xe)
  Constant7/1 -> vektor um eulerwinkel drehen rc/5(ye)
  Constant8/1 -> vektor um eulerwinkel drehen rc/6(ze)
  Constant9/1 -> vektor um eulerwinkel drehen rd/4(xe)
  Constant10/1 -> vektor um eulerwinkel drehen rd/5(ye)
  Constant11/1 -> vektor um eulerwinkel drehen rd/6(ze)

== system regler/Regelkreis/Motor/Moment Subsystem/n<1 ==
  Action Port : ActionPort  ActionType=else
  Constant : Constant  Value=0
  M : Outport  InitialOutput=[0]
  wires:
  Constant/1 -> M/1

== system regler/Regelkreis/Motor/Moment Subsystem/n>0 ==
  n : Inport
  Action Port : ActionPort  ActionType=then
  Add : Sum
  Constant : Constant  Value=cm
  Gain : Gain  Gain=mm
  M : Outport
  wires:
  Gain/1 -> Add/1
  Constant/1 -> Add/2
  Add/1 -> M/1
  n/1 -> Gain/1

== system regler/Regelkreis/Motor/Moment Subsystem1/n<1 ==
  Action Port : ActionPort  ActionType=else
  Constant : Constant  Value=0
  M : Outport  InitialOutput=[0]
  wires:
  Constant/1 -> M/1

== system regler/Regelkreis/Motor/Moment Subsystem1/n>0 ==
  n : Inport
  Action Port : ActionPort  ActionType=then
  Add : Sum
  Constant : Constant  Value=cm
  Gain : Gain  Gain=mm
  M : Outport
  wires:
  n/1 -> Gain/1
  Add/1 -> M/1
  Constant/1 -> Add/2
  Gain/1 -> Add/1

== system regler/Regelkreis/Motor/Moment Subsystem2/n<1 ==
  Action Port : ActionPort  ActionType=else
  Constant : Constant  Value=0
  M : Outport  InitialOutput=[0]
  wires:
  Constant/1 -> M/1

== system regler/Regelkreis/Motor/Moment Subsystem2/n>0 ==
  n : Inport
  Action Port : ActionPort  ActionType=then
  Add : Sum
  Constant : Constant  Value=cm
  Gain : Gain  Gain=mm
  M : Outport
  wires:
  Gain/1 -> Add/1
  Constant/1 -> Add/2
  Add/1 -> M/1
  n/1 -> Gain/1

== system regler/Regelkreis/Motor/Moment Subsystem3/n<1 ==
  Action Port : ActionPort  ActionType=else
  Constant : Constant  Value=0
  M : Outport  InitialOutput=[0]
  wires:
  Constant/1 -> M/1

== system regler/Regelkreis/Motor/Moment Subsystem3/n>0 ==
  n : Inport
  Action Port : ActionPort  ActionType=then
  Add : Sum
  Constant : Constant  Value=cm
  Gain : Gain  Gain=mm
  M : Outport
  wires:
  n/1 -> Gain/1
  Add/1 -> M/1
  Constant/1 -> Add/2
  Gain/1 -> Add/1

== system regler/Regelkreis/Schubverteilung/Begrenzung groeßer Null/If Action Subsystem ==
  In1 : Inport
  Action Port : ActionPort  ActionType=then
  Out1 : Outport
  wires:
  In1/1 -> Out1/1

== system regler/Regelkreis/Schubverteilung/Begrenzung groeßer Null/If Action Subsystem1 ==
  Action Port : ActionPort  ActionType=else
  Constant : Constant  Value=0
  Out1 : Outport
  wires:
  Constant/1 -> Out1/1

== system regler/Regelkreis/Schubverteilung/Begrenzung groeßer Null1/If Action Subsystem ==
  In1 : Inport
  Action Port : ActionPort  ActionType=then
  Out1 : Outport
  wires:
  In1/1 -> Out1/1

== system regler/Regelkreis/Schubverteilung/Begrenzung groeßer Null1/If Action Subsystem1 ==
  Action Port : ActionPort  ActionType=else
  Constant : Constant  Value=0
  Out1 : Outport
  wires:
  Constant/1 -> Out1/1

== system regler/Regelkreis/Schubverteilung/Begrenzung groeßer Null2/If Action Subsystem ==
  In1 : Inport
  Action Port : ActionPort  ActionType=then
  Out1 : Outport
  wires:
  In1/1 -> Out1/1

== system regler/Regelkreis/Schubverteilung/Begrenzung groeßer Null2/If Action Subsystem1 ==
  Action Port : ActionPort  ActionType=else
  Constant : Constant  Value=0
  Out1 : Outport
  wires:
  Constant/1 -> Out1/1

== system regler/Regelkreis/Schubverteilung/Begrenzung groeßer Null3/If Action Subsystem ==
  In1 : Inport
  Action Port : ActionPort  ActionType=then
  Out1 : Outport
  wires:
  In1/1 -> Out1/1

== system regler/Regelkreis/Schubverteilung/Begrenzung groeßer Null3/If Action Subsystem1 ==
  Action Port : ActionPort  ActionType=else
  Constant : Constant  Value=0
  Out1 : Outport
  wires:
  Constant/1 -> Out1/1

== matlab function Regelkreis/Chassis/Gewichtskraft//Moment/chassis drehen/vektor um eulerwinkel drehen rc ==
  data: gier input double; xa output double; nick input double; roll input double; xe input double; ye input double; ze input double; ya output double; za output double
function [xa, ya, za] = fcn(gier, nick, roll, xe, ye, ze)
ve=[xe;
    ye;
    ze];

rot_roll=[1 0 0;
         0 cos(roll) sin(roll);
         0 -sin(roll) cos(roll)];
     
rot_nick=[cos(nick) 0 -sin(nick)
         0 1 0;
         sin(nick) 0 cos(nick)];
rot_gier=[cos(gier) sin(gier) 0;
         -sin(gier) cos(gier) 0;
         0 0 1];
     
va=(rot_roll*rot_nick*rot_gier)*ve;
xa=va(1);
ya=va(2);
za=va(3);

== matlab function Regelkreis/Chassis/Gewichtskraft//Moment/chassis drehen/vektor um eulerwinkel drehen rb ==
  data: gier input double; xa output double; nick input double; roll input double; xe input double; ye input double; ze input double; ya output double; za output double
function [xa, ya, za] = fcn(gier, nick, roll, xe, ye, ze)
ve=[xe;
    ye;
    ze];

rot_roll=[1 0 0;
         0 cos(roll) sin(roll);
         0 -sin(roll) cos(roll)];
     
rot_nick=[cos(nick) 0 -sin(nick)
         0 1 0;
         sin(nick) 0 cos(nick)];
rot_gier=[cos(gier) sin(gier) 0;
         -sin(gier) cos(gier) 0;
         0 0 1];
     
va=(rot_roll*rot_nick*rot_gier)*ve;
xa=va(1);
ya=va(2);
za=va(3);

== matlab function Regelkreis/Chassis/Gewichtskraft//Moment/chassis drehen/vektor um eulerwinkel drehen ra ==
  data: gier input double; xa output double; nick input double; roll input double; xe input double; ye input double; ze input double; ya output double; za output double
function [xa,ya,za] = fcn(gier, nick, roll, xe, ye, ze)
%#codegen

ve=[xe;
    ye;
    ze];

rot_roll=[1 0 0;
         0 cos(roll) sin(roll);
         0 -sin(roll) cos(roll)];
     
rot_nick=[cos(nick) 0 -sin(nick)
         0 1 0;
         sin(nick) 0 cos(nick)];
rot_gier=[cos(gier) sin(gier) 0;
         -sin(gier) cos(gier) 0;
         0 0 1];
     
va=(rot_roll*rot_nick*rot_gier)*ve;
xa=va(1);
ya=va(2);
za=va(3);

== matlab function Regelkreis/Chassis/Gewichtskraft//Moment/chassis drehen/vektor um eulerwinkel drehen rd ==
  data: gier input double; xa output double; nick input double; roll input double; xe input double; ye input double; ze input double; ya output double; za output double
function [xa, ya, za] = fcn(gier, nick, roll, xe, ye, ze)
ve=[xe;
    ye;
    ze];

rot_roll=[1 0 0;
         0 cos(roll) sin(roll);
         0 -sin(roll) cos(roll)];
     
rot_nick=[cos(nick) 0 -sin(nick)
         0 1 0;
         sin(nick) 0 cos(nick)];
rot_gier=[cos(gier) sin(gier) 0;
         -sin(gier) cos(gier) 0;
         0 0 1];
     
va=(rot_roll*rot_nick*rot_gier)*ve;
xa=va(1);
ya=va(2);
za=va(3);

== matlab function Regelkreis/Chassis/Gewichtskraft//Moment/Einheitskraftvektor drehen/vektor um eulerwinkel drehen ra ==
  data: gier input double; xa output double; nick input double; roll input double; xe input double; ye input double; ze input double; ya output double; za output double
function [xa,ya,za] = fcn(gier, nick, roll, xe, ye, ze)
%#codegen

ve=[xe;
    ye;
    ze];

rot_roll=[1 0 0;
         0 cos(roll) sin(roll);
         0 -sin(roll) cos(roll)];
     
rot_nick=[cos(nick) 0 -sin(nick)
         0 1 0;
         sin(nick) 0 cos(nick)];
rot_gier=[cos(gier) sin(gier) 0;
         -sin(gier) cos(gier) 0;
         0 0 1];
     
va=(rot_roll*rot_nick*rot_gier)*ve;
xa=va(1);
ya=va(2);
za=va(3);
